simulink model "Proyecto_Motor_Lazo_Abierto"  (R2017b)
settings: Solver=VariableStepAuto  StartTime=0.0  StopTime=1  MaxStep=1e-4  RelTol=1e-3
values from neighbouring files (symbols this model uses):
  Ts = 2e-3    (= 0.002)    [Ploteo_Datos.m]
undefined symbols (not defined in the file or in its folder): Jm, Ke, Kt, La, Ra, Vcc
libraries: powerlib x17, powerlib_meascontrol x1
settings Model: Creator=ezema  LastModifiedBy=ezema

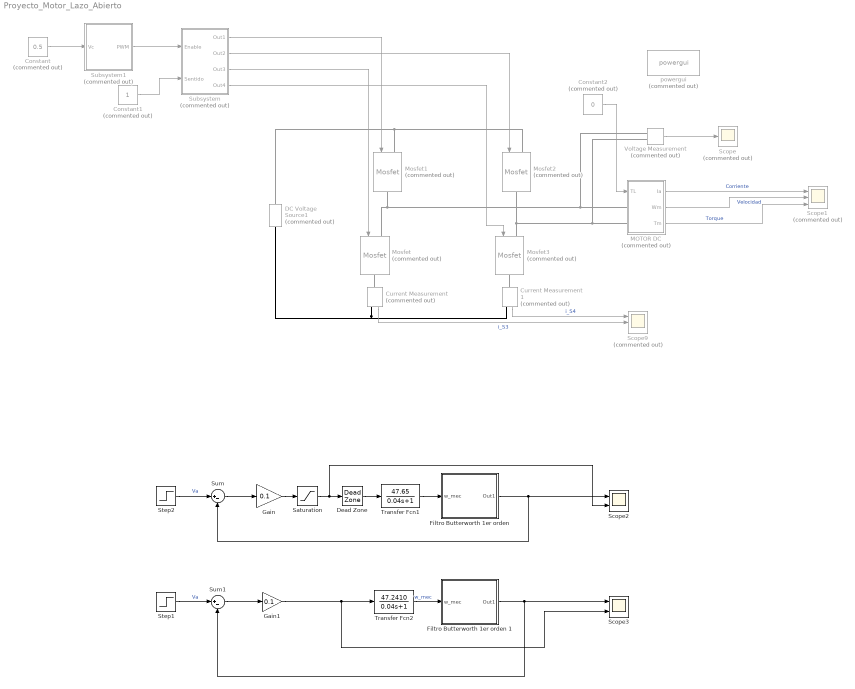
== system Proyecto_Motor_Lazo_Abierto ==
  Constant : Constant  Commented=on  Value=0.5
  Constant1 : Constant  Commented=on
  Constant2 : Constant  Commented=on  Value=0
  Current Measurement : powerlib/Measurements/Current Measurement  Commented=on  PhasorSimulation=off  OutputType=Complex  PSBequivalent=0
  Current Measurement1 : powerlib/Measurements/Current Measurement  Commented=on  PhasorSimulation=off  OutputType=Complex  PSBequivalent=0
  DC Voltage Source1 : powerlib/Electrical Sources/DC Voltage Source  Commented=on  Amplitude=Vcc  Measurements=None
  Dead Zone : DeadZone  LowerValue=-8.512  UpperValue=8.512  SaturateOnIntegerOverflow=on
  "Filtro Butterworth 1er orden " : Subsystem
  Filtro Butterworth 1er orden 1 : Subsystem
  Gain : Gain  Gain=0.1
  Gain1 : Gain  Gain=0.1
  "MOTOR DC " : Subsystem  Commented=on
  Mosfet{,1..3} (4 alike) : powerlib/Power Electronics/Mosfet  Commented=on  Ron=0  Lon=0  Rd=0  Vfd=0  IC=0  Rs=inf  Cs=inf  Measurements=off
  Saturation : Saturate  UpperLimit=17  LowerLimit=8.5
  Scope : Scope  Commented=on
  Scope1 : Scope  Commented=on  NumInputPorts=3
  Scope2 : Scope  NumInputPorts=2
  Scope3 : Scope  NumInputPorts=2
  Scope9 : Scope  Commented=on  NumInputPorts=3
  Step1 : Step  Time=0  After=200  SampleTime=0
  Step2 : Step  Time=0  After=200  SampleTime=0
  Subsystem : Subsystem  Commented=on
  Subsystem1 : Subsystem  Commented=on
  Sum : Sum  Inputs=|+-
  Sum1 : Sum  Inputs=|+-
  Transfer Fcn1 : TransferFcn  Numerator=[47.65]  Denominator=[0.04 1]
  Transfer Fcn2 : TransferFcn  Numerator=[47.2410]  Denominator=[0.04 1]
  Voltage Measurement : powerlib/Measurements/Voltage Measurement  Commented=on  PhasorSimulation=off  OutputType=Complex  PSBequivalent=0
  powergui : powerlib/powergui  Priority=1  Commented=on  SimulationMode=Continuous  SampleTime=50e-6  frequency=60  Iterations=50  frequencyindice=0  Pbase=100e6  ErrMax=1e-4  UnitsV=kV  UnitsW=MW  buscounter=0  FunctionMessages=off  echomessages=off  EnableUseOfTLC=off  CurrentSourceSwitches=off  DisableSnubberDevices=off  DisableRonSwitches=off  DisableVfSwitches=off  DisplayEquations=off  SolverType=Tustin/Backward Euler (TBE)  Interpol=off  ExternalGateDelay=off  methode=off  Ts=100  x0status=blocks  SPID=on  SwTol=0  HookPort=off  RestoreLinks=warning  ResistiveCurrentMeasurement=off  Frange=[0:2:500]  Ylog=off  Xlog=on  ShowGrid=off  save=off  variable=ZData  structure=0  ZoomFFT=off  StartTime=0.0  cycles=1  DisplayStyle=1  fundamental=60  FreqAxis=off  MaxFrequency=1000  frequencyindicesteady=1  RmsSteady=1  display=off
  wires:
  Voltage Measurement/1 -> Scope/1
  Current Measurement1/1 -> Scope9/1  "i_S4"
  Current Measurement/1 -> Scope9/2  "i_S3"
  "MOTOR DC "/3(Tm) -> Scope1/3  "Torque"
  "MOTOR DC "/2(Wm) -> Scope1/2  "Velocidad"
  Constant2/1 -> "MOTOR DC "/1(TL)
  "MOTOR DC "/1(Ia) -> Scope1/1  "Corriente"
  Subsystem/1(Out1) -> Mosfet1/1
  Subsystem/2(Out2) -> Mosfet2/1
  Subsystem/3("Out3 ") -> Mosfet/1
  Subsystem/4("Out4 ") -> Mosfet3/1
  Subsystem1/1("PWM ") -> Subsystem/1(Enable)
  Constant1/1 -> Subsystem/2(Sentido)
  Constant/1 -> Subsystem1/1(Vc)
  Step2/1 -> Sum/1  "Va"
  Sum/1 -> Gain/1
  Gain/1 -> Saturation/1
  Dead Zone/1 -> Transfer Fcn1/1
  Step1/1 -> Sum1/1  "Va"
  Gain1/1 -> Scope3/2, Transfer Fcn2/1
  Sum1/1 -> Gain1/1
  Transfer Fcn1/1 -> "Filtro Butterworth 1er orden "/1(w_mec)
  "Filtro Butterworth 1er orden "/1(Out1) -> Sum/2, Scope2/1
  Saturation/1 -> Scope2/2, Dead Zone/1
  Transfer Fcn2/1 -> Filtro Butterworth 1er orden 1/1(w_mec)  "w_mec"
  Filtro Butterworth 1er orden 1/1(Out1) -> Sum1/2, Scope3/1
  connections:
  "MOTOR DC "/LConn2 -- Mosfet2/RConn1 -- Mosfet3/LConn1 -- Voltage Measurement/LConn2
  Current Measurement/RConn1 -- Current Measurement1/RConn1 -- DC Voltage Source1/LConn1
  "MOTOR DC "/LConn1 -- Mosfet1/RConn1 -- Mosfet/LConn1 -- Voltage Measurement/LConn1
  DC Voltage Source1/RConn1 -- Mosfet1/LConn1 -- Mosfet2/LConn1
  Current Measurement1/LConn1 -- Mosfet3/RConn1
  Current Measurement/LConn1 -- Mosfet/RConn1

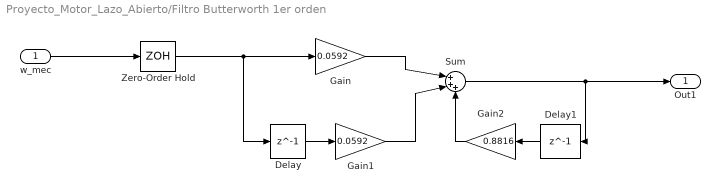
== system Proyecto_Motor_Lazo_Abierto/Filtro Butterworth 1er orden  ==
  w_mec : Inport
  Delay : Delay  DelayLength=1  SampleTime=Ts
  Delay1 : Delay  DelayLength=1  SampleTime=Ts
  Gain : Gain  Gain=0.0592
  Gain1 : Gain  Gain=0.0592
  Gain2 : Gain  Gain=0.8816
  Sum : Sum  Inputs=|+++
  Zero-Order Hold : ZeroOrderHold  SampleTime=Ts
  Out1 : Outport
  wires:
  Gain2/1 -> Sum/3
  Delay1/1 -> Gain2/1
  Gain/1 -> Sum/1
  Delay/1 -> Gain1/1
  Zero-Order Hold/1 -> Gain/1, Delay/1
  Sum/1 -> Out1/1, Delay1/1
  Gain1/1 -> Sum/2
  w_mec/1 -> Zero-Order Hold/1

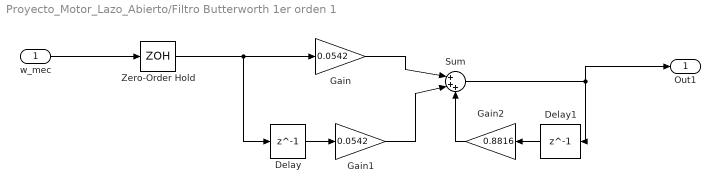
== system Proyecto_Motor_Lazo_Abierto/Filtro Butterworth 1er orden 1 ==
  w_mec : Inport
  Delay : Delay  DelayLength=1  SampleTime=Ts
  Delay1 : Delay  DelayLength=1  SampleTime=Ts
  Gain : Gain  Gain=0.0542
  Gain1 : Gain  Gain=0.0542
  Gain2 : Gain  Gain=0.8816
  Sum : Sum  Inputs=|+++
  Zero-Order Hold : ZeroOrderHold  SampleTime=Ts
  Out1 : Outport
  wires:
  Gain2/1 -> Sum/3
  Delay1/1 -> Gain2/1
  Gain/1 -> Sum/1
  Delay/1 -> Gain1/1
  Zero-Order Hold/1 -> Gain/1, Delay/1
  Sum/1 -> Out1/1, Delay1/1
  Gain1/1 -> Sum/2
  w_mec/1 -> Zero-Order Hold/1

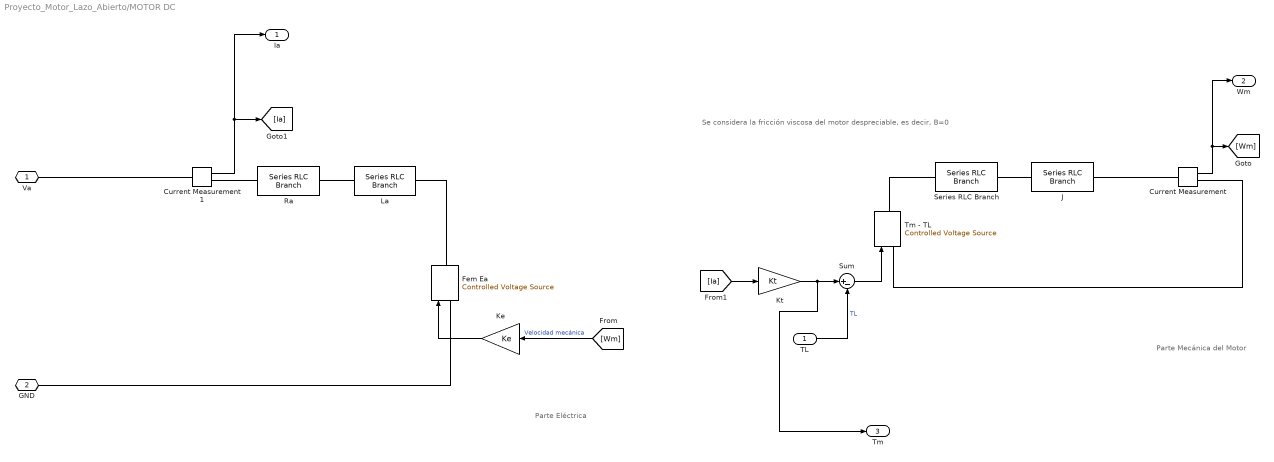
== system Proyecto_Motor_Lazo_Abierto/MOTOR DC  ==
  note: Se considera la fricción viscosa del motor despreciable, es decir, B=0
  note: Parte Eléctrica
  note: Parte Mecánica del Motor
  TL : Inport
  " Fem Ea" : powerlib/Electrical Sources/Controlled Voltage Source  Initialize=on  Source_Type=DC  Amplitude=0  Phase=0  Frequency=0  Measurements=None
  " Tm - TL" : powerlib/Electrical Sources/Controlled Voltage Source  Initialize=on  Source_Type=DC  Amplitude=0  Phase=0  Frequency=0  Measurements=None
  Current Measurement : powerlib/Measurements/Current Measurement  PhasorSimulation=off  OutputType=Complex  PSBequivalent=0
  Current Measurement1 : powerlib/Measurements/Current Measurement  PhasorSimulation=off  OutputType=Complex  PSBequivalent=0
  J : powerlib/Elements/Series RLC Branch  LConnTagsString=__new0  RConnTagsString=__new0  BranchType=L  Resistance=1  Inductance=Jm  SetiL0=off  InitialCurrent=0  Capacitance=1e-6  Setx0=off  InitialVoltage=0  Measurements=None
  Ke : Gain  Gain=Ke
  Kt : Gain  Gain=Kt
  La : powerlib/Elements/Series RLC Branch  LConnTagsString=__new0  RConnTagsString=__new0  BranchType=L  Resistance=1  Inductance=La  SetiL0=off  InitialCurrent=0  Capacitance=1e-6  Setx0=off  InitialVoltage=0  Measurements=None
  Ra : powerlib/Elements/Series RLC Branch  LConnTagsString=__new0  RConnTagsString=__new0  BranchType=R  Resistance=Ra  Inductance=1e-3  SetiL0=off  InitialCurrent=0  Capacitance=1e-6  Setx0=off  InitialVoltage=0  Measurements=None
  Series RLC Branch : powerlib/Elements/Series RLC Branch  LConnTagsString=__new0  RConnTagsString=__new0  BranchType=R  Resistance=1e-4  Inductance=1e-3  SetiL0=off  InitialCurrent=0  Capacitance=1e-6  Setx0=off  InitialVoltage=0  Measurements=None
  Sum : Sum  Inputs=|+-
  Va : PMIOPort  Port=1  Side=Left
  GND : PMIOPort  Port=2  Side=Left
  Ia : Outport
  Wm : Outport  Port=2
  Tm : Outport  Port=3
  wires:
  Sum/1 -> " Tm - TL"/1
  TL/1 -> Sum/2  "TL"
  [Wm] -> Ke/1  "Velocidad mecánica"
  Current Measurement1/1 -> Ia/1, [Ia]
  Kt/1 -> Tm/1, Sum/1
  Ke/1 -> " Fem Ea"/1
  [Ia] -> Kt/1
  Current Measurement/1 -> Wm/1, [Wm]
  connections:
  " Fem Ea"/RConn1 -- La/RConn1
  Current Measurement/RConn1 -- " Tm - TL"/LConn1
  Current Measurement1/RConn1 -- Ra/LConn1
  La/LConn1 -- Ra/RConn1
  Current Measurement/LConn1 -- J/RConn1
  Va/RConn1 -- Current Measurement1/LConn1
  " Fem Ea"/LConn1 -- GND/RConn1
  Series RLC Branch/RConn1 -- J/LConn1
  Series RLC Branch/LConn1 -- " Tm - TL"/RConn1

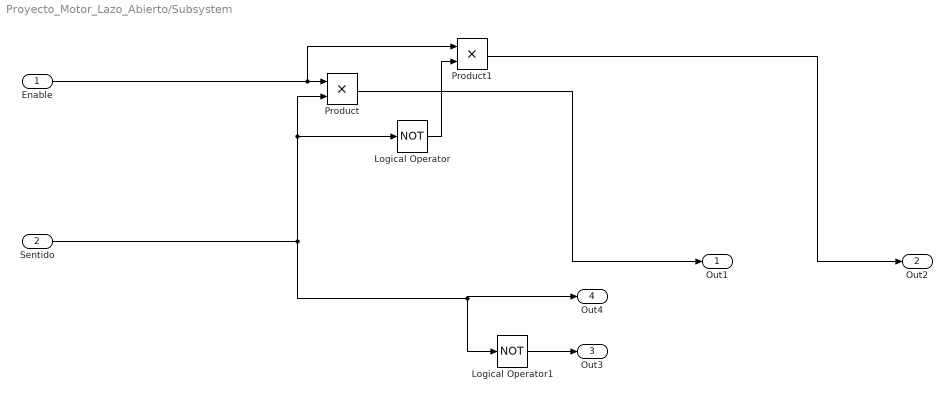
== system Proyecto_Motor_Lazo_Abierto/Subsystem ==
  Enable : Inport
  Sentido : Inport  Port=2
  Logical Operator : Logic  Operator=NOT  AllPortsSameDT=off  OutDataTypeStr=boolean
  Logical Operator1 : Logic  Operator=NOT  AllPortsSameDT=off  OutDataTypeStr=boolean
  Product : Product
  Product1 : Product
  Out1 : Outport
  Out2 : Outport  Port=2
  "Out3 " : Outport  Port=3
  "Out4 " : Outport  Port=4
  wires:
  Logical Operator/1 -> Product1/2
  Enable/1 -> Product1/1, Product/1
  Product/1 -> Out1/1
  Product1/1 -> Out2/1
  Sentido/1 -> Logical Operator1/1, "Out4 "/1, Logical Operator/1, Product/2
  Logical Operator1/1 -> "Out3 "/1

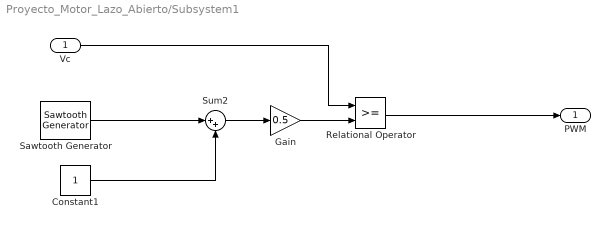
== system Proyecto_Motor_Lazo_Abierto/Subsystem1 ==
  Vc : Inport
  Constant1 : Constant
  Gain : Gain  Gain=0.5
  Relational Operator : RelationalOperator  OutDataTypeStr=boolean  RndMeth=Round
  Sawtooth Generator : powerlib_meascontrol/Pulse & Signal Generators/Sawtooth Generator  Freq=5e3  Phase=0  Ts=0
      settings: SourceProductName=Simscape Power Systems
  Sum2 : Sum  Inputs=|++
  "PWM " : Outport
  wires:
  Vc/1 -> Relational Operator/1
  Relational Operator/1 -> "PWM "/1
  Constant1/1 -> Sum2/2
  Sawtooth Generator/1 -> Sum2/1
  Gain/1 -> Relational Operator/2
  Sum2/1 -> Gain/1
